simulink model "Example_1_Open"  (Simulink 8.3)
settings: Solver=ode45  StartTime=0.0  StopTime=50  RelTol=1e-3
libraries: simulink x1
settings Model: Creator=NeuControl  LastModifiedBy=Li Jinghao
settings DataIOCC: SignalLoggingSaveFormat=Dataset
settings DebuggingCC: UnderspecifiedInitializationDetection=Simplified  StateNameClashWarn=none
settings GRTTargetCC: CombineOutputUpdateFcns=on  GRTInterface=off

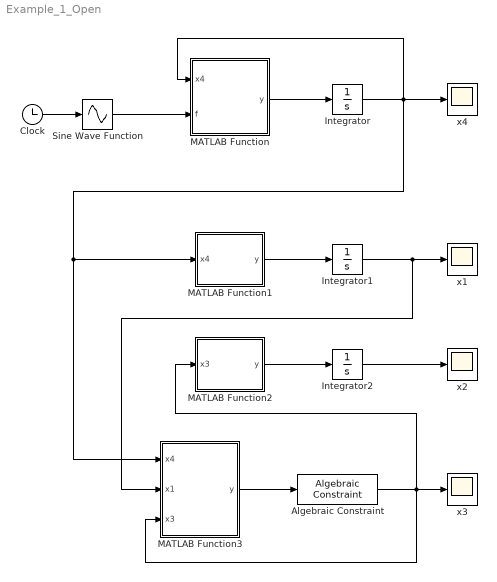
== system Example_1_Open ==
  Algebraic Constraint : simulink/Math Operations/Algebraic Constraint  z0=0
  Clock : Clock
  Integrator : Integrator  InitialCondition=0.5*pi
  Integrator1 : Integrator  InitialCondition=0.3*pi
  Integrator2 : Integrator  InitialCondition=-5
  MATLAB Function : MATLAB Function  TreatAsAtomicUnit=on
  MATLAB Function1 : MATLAB Function  TreatAsAtomicUnit=on
  MATLAB Function2 : MATLAB Function  TreatAsAtomicUnit=on
  MATLAB Function3 : MATLAB Function  TreatAsAtomicUnit=on
  Sine Wave Function : Sin  TimeSource=Use external signal  SampleTime=0
  x{1..4} (4 alike) : Scope
      x1 settings: SaveName=x1
      x2 settings: SaveName=x2
      x3 settings: SaveName=x3
      x4 settings: SaveName=x4
  wires:
  MATLAB Function/1(y) -> Integrator/1
  Integrator/1 -> MATLAB Function3/1(x4), MATLAB Function1/1(x4), MATLAB Function/1(x4), x4/1
  Sine Wave Function/1 -> MATLAB Function/2(f)
  Clock/1 -> Sine Wave Function/1
  MATLAB Function1/1(y) -> Integrator1/1
  Integrator1/1 -> MATLAB Function3/2(x1), x1/1
  MATLAB Function2/1(y) -> Integrator2/1
  Integrator2/1 -> x2/1
  Algebraic Constraint/1 -> MATLAB Function3/3(x3), MATLAB Function2/1(x3), x3/1
  MATLAB Function3/1(y) -> Algebraic Constraint/1

== matlab function MATLAB Function1 ==
  data: x4 input double; y output double
function y = fcn(x4)
%#codegen

Ll=5.5;
v=-1;
bt=2;
t0=0.5;

y = v*bt/(Ll*t0)*x4;

== matlab function MATLAB Function ==
  data: x4 input double; y output double; f input double
function y = fcn(x4,f)
%#codegen

l=2.8;
Ll=5.5;
v=-1;
bt=2;
t0=0.5;


y = -v*bt/(Ll*t0)*x4+v*bt/(l*t0)*f;

== matlab function MATLAB Function2 ==
  data: x3 input double; y output double
function y = fcn(x3)
%#codegen

v=-1;
bt=2;
t0=0.5;

y = v*bt/t0*x3;

== matlab function MATLAB Function3 ==
  data: x4 input double; x1 input double; x3 input double; y output double
function y = fcn(x4,x1,x3)
%#codegen

Ll=5.5;
v=-1;
bt=2;

y = sin(x1+v*bt/(2*Ll)*x4)-x3;
